simulink model "SF018A_EotProtn"  (R2013b)
settings: Solver=FixedStepDiscrete  SolverMode=SingleTasking  StartTime=0.0  StopTime=0.002  FixedStep=.002  RelTol=1e-3
undefined symbols (not defined in the file): ALLSPDDAMPG_CNT_U08, ALLSPDGAIN_CNT_U08, ARCHGLBPRM_2MILLISEC_SEC_F32, DISTLPFILFRQ_HZ_F32, EOTDAMPGLOLIM_MOTNWTMTR_F32, EOTGAINHILIM_ULS_F32, EotProtnActvRegnBypMaxThd, EotProtnDampgSlew, EotProtnDampgVehSpdTbl, EotProtnDeltaTqThd, EotProtnDftPosn, EotProtnEntrGainVehSpdTbl, EotProtnEntrGainX, EotProtnEntrStLpFilFrq, EotProtnExitDampgY, EotProtnExitStLpFilFrq, EotProtnHwAgGain, EotProtnHwAgMax, EotProtnHwAgMin, EotProtnHwDegDampgX, EotProtnMotSpdIncptSca, EotProtnMotSpdIncptX, EotProtnMotSpdIncptY, EotProtnMotVelGain, EotProtnNormDampgY, EotProtnPosnRampStep, EotProtnRackTrvlLimrAuthyThd, EotProtnRackTrvlLimrAuthyThdLimd, EotProtnRackTrvlLimrEna, EotProtnRackTrvlLimrRng, EotProtnRackTrvlLimrRngLimd, EotProtnRackTrvlLimrVehSpdThd, EotProtnRunEotVelImpctAndSoftEndStop, EotProtnSoftEndStopAuthyThd, EotProtnSoftEndStopEna, EotProtnSoftEndStopVehSpdThd, FIRSTPTDAMPG_CNT_U08, LASTPTGAIN_CNT_U08, SOFTENDSTOPSTDI_CNT_U08, SOFTENDSTOPSTENTR_CNT_U08, SOFTENDSTOPSTEXIT_CNT_U08, SOFTENDSTOPSTNORM_CNT_U08, SYSGLBPRM_MOTTQCMDHILIM_MOTNWTMTR_F32, ZEROMOTTQCMD_MOTNWTMTR_F32
libraries: NxtrAbslt x16, FloatToFixd x14, FixdToFloat x6, Fil x5, NxtrLim x5, simulink x4, NxtrMax x4, LnrIntrpnDyn x3, NxtrSign x2, BilnrIntrpnMplXDyn x2, BilnrIntrpnMplX x1, LnrIntrpn x1
(part 4 of 5)

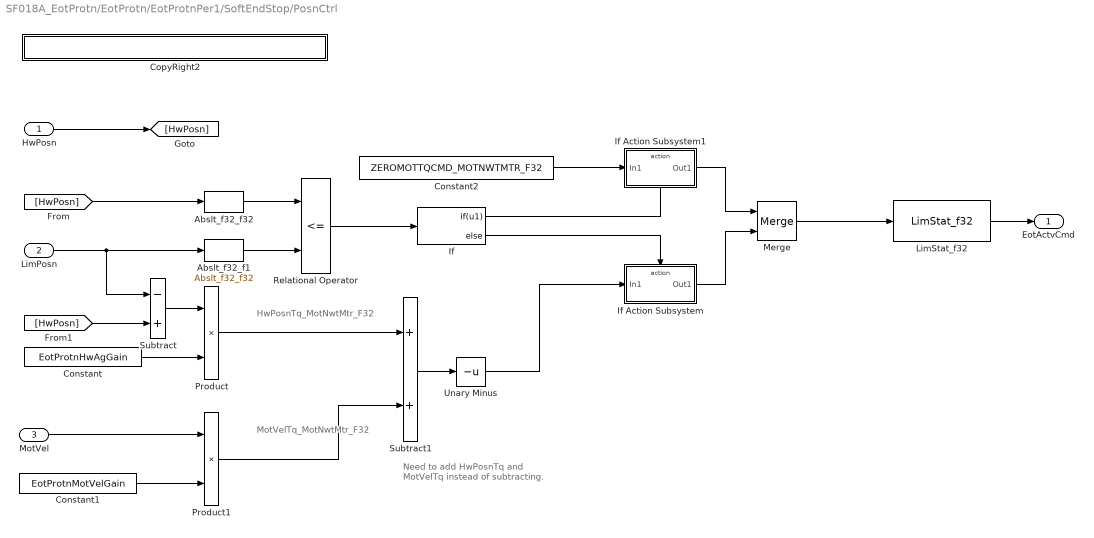
== system SF018A_EotProtn/EotProtn/EotProtnPer1/SoftEndStop/PosnCtrl ==
  note: Need to add HwPosnTq and
      | MotVelTq instead of subtracting.
  note: HwPosnTq_MotNwtMtr_F32
  note: MotVelTq_MotNwtMtr_F32
  HwPosn : Inport
  LimPosn : Inport  Port=2
  MotVel : Inport  Port=3
  Abslt_f32_f1 : NxtrAbslt/Abslt_f32_f32  SFunctionSpec=single y1 = Abslt_f32_f32(single u1)
      settings: AttributesFormatString=%<Name>
  Abslt_f32_f32 : NxtrAbslt/Abslt_f32_f32  SFunctionSpec=single y1 = Abslt_f32_f32(single u1)
      settings: AttributesFormatString=%<Name>
  Constant : Constant  Value=EotProtnHwAgGain
  Constant1 : Constant  Value=EotProtnMotVelGain
  Constant2 : Constant  RequirementInfo={'linktype_rmi_doors' '0000ba56 (/E-STEER Core/SubSystem Specifications/Application Functions/SF018A End-of-Travel Actuator Management- EOT Impact and Soft Stops)' '#SF018A_118' 'true' 'REQ: SF018A_118' '' } %GIDa_3d57071b_fdcd_4c59_a01b_b9a326557455  Value=ZEROMOTTQCMD_MOTNWTMTR_F32
  CopyRight2 : Subsystem  Description=|  mask(Copyright Information){none=on}
      | Copyright info block.                                               
      |                                                                     
      | Place copyright information at the top of every subsystem in design.
      mask prompts: none "No parameters"
      mask help: Place copyright information at the top of every subsystem in design.
      mask Display:
      | NxtrConf = 'Nexteer Confidential';
      | 
      | sys = bdroot; %handle for the current model ("system")
      | first = get_param(sys,'Created');
      | if(isempty(first))
      |     first = datestr(now,'yyyy');
      | else
      |     first = first(end-3:end);  %year is last four digits
      | end
      | 
      | last = get_param(sys,'LastModifiedDate');
      | if isempty(last)
      |     last = datestr(now,'yyyy');
      | else
      |     last = last(end-3:end);
      | end
      | 
      | if strcmp(first,last)
      |     fprintf('%s -- Copyright %s Nexteer',NxtrConf,first)
      | else
      |     fprintf('%s -- %s%s- %s Nexteer',NxtrConf,char(169),first,last)
      | end
  If : If  RequirementInfo={'linktype_rmi_doors' '0000ba56 (/E-STEER Core/SubSystem Specifications/Application Functions/SF018A End-of-Travel Actuator Management- EOT Impact and Soft Stops)' '#SF018A_118' 'true' 'REQ: SF018A_118' '' } %GIDa_eb767372_f633_4e49_a326_b612579dcde1  IfExpression=u1
  If Action Subsystem : Subsystem  RequirementInfo={'linktype_rmi_doors' '0000ba56 (/E-STEER Core/SubSystem Specifications/Application Functions/SF018A End-of-Travel Actuator Management- EOT Impact and Soft Stops)' '#SF018A_118' 'true' 'REQ: SF018A_118' '' } %GIDa_35741698_416e_4048_a750_0a2756a8727b  TreatAsAtomicUnit=on
  If Action Subsystem1 : Subsystem  RequirementInfo={'linktype_rmi_doors' '0000ba56 (/E-STEER Core/SubSystem Specifications/Application Functions/SF018A End-of-Travel Actuator Management- EOT Impact and Soft Stops)' '#SF018A_118' 'true' 'REQ: SF018A_118' '' } %GIDa_3f03eff5_f878_4981_ae49_8a66d8cca778  TreatAsAtomicUnit=on
  LimStat_f32 : NxtrLim/LimStat_f32  RequirementInfo={'linktype_rmi_doors' '0000ba56 (/E-STEER Core/SubSystem Specifications/Application Functions/SF018A End-of-Travel Actuator Management- EOT Impact and Soft Stops)' '#SF018A_115' 'true' 'REQ: SF018A_115' '' } %GIDa_f450d0e0_b743_4f7d_a6bc_c122e939de08  LoLim=SYSGLBPRM_MOTTQCMDLOLIM_MOTNWTMTR_F32  HiLim=SYSGLBPRM_MOTTQCMDHILIM_MOTNWTMTR_F32
      settings: AttributesFormatString=|
      | Low Limit: %<LoLim>
      | High Limit:%<HiLim>
  Merge : Merge  RequirementInfo={'linktype_rmi_doors' '0000ba56 (/E-STEER Core/SubSystem Specifications/Application Functions/SF018A End-of-Travel Actuator Management- EOT Impact and Soft Stops)' '#SF018A_118' 'true' 'REQ: SF018A_118' '' } %GIDa_35b0fcf4_10cf_4d00_afb1_7de2ceba647a
  Product : Product  RequirementInfo={'linktype_rmi_doors' '0000ba56 (/E-STEER Core/SubSystem Specifications/Application Functions/SF018A End-of-Travel Actuator Management- EOT Impact and Soft Stops)' '#SF018A_115' 'true' 'REQ: SF018A_115' '' } %GIDa_75e8deb4_4dc3_4dee_b8fd_971ee3dd6133
  Product1 : Product  RequirementInfo={'linktype_rmi_doors' '0000ba56 (/E-STEER Core/SubSystem Specifications/Application Functions/SF018A End-of-Travel Actuator Management- EOT Impact and Soft Stops)' '#SF018A_115' 'true' 'REQ: SF018A_115' '' } %GIDa_7846ba9c_06f8_474a_b2f4_81c28a29a3d7
  Relational Operator : RelationalOperator  RequirementInfo={'linktype_rmi_doors' '0000ba56 (/E-STEER Core/SubSystem Specifications/Application Functions/SF018A End-of-Travel Actuator Management- EOT Impact and Soft Stops)' '#SF018A_118' 'true' 'REQ: SF018A_118' '' } %GIDa_f3de5d6e_d215_4d21_9e68_558719ac5ade  Operator=<=  OutDataTypeStr=boolean
  Subtract : Sum  RequirementInfo={'linktype_rmi_doors' '0000ba56 (/E-STEER Core/SubSystem Specifications/Application Functions/SF018A End-of-Travel Actuator Management- EOT Impact and Soft Stops)' '#SF018A_115' 'true' 'REQ: SF018A_115' '' } %GIDa_15a4990c_45d6_482c_b0b5_8f5c16105016  Inputs=-+
  Subtract1 : Sum  RequirementInfo={'linktype_rmi_doors' '0000ba56 (/E-STEER Core/SubSystem Specifications/Application Functions/SF018A End-of-Travel Actuator Management- EOT Impact and Soft Stops)' '#SF018A_116' 'true' 'REQ: SF018A_116' '' ; 'linktype_rmi_doors' '0000ba56 (/E-STEER Core/SubSystem Specifications/Application Functions/SF018A End-of-Travel Actuator Management- EOT Impact and Soft Stops)' '#SF018A_117' 'true' 'REQ: SF018A_117' '' } %GIDa_cd110dc1_ef6c_4228_8a84_7b55c0e467bf
  Unary Minus : UnaryMinus
  EotActvCmd : Outport
  wires:
  Unary Minus/1 -> If Action Subsystem/1(In1)
  LimStat_f32/1 -> EotActvCmd/1
  Merge/1 -> LimStat_f32/1
  If Action Subsystem/1(Out1) -> Merge/2
  If Action Subsystem1/1(Out1) -> Merge/1
  Constant2/1 -> If Action Subsystem1/1(In1)
  If/1 -> If Action Subsystem1/Action
  If/2 -> If Action Subsystem/Action
  Subtract1/1 -> Unary Minus/1
  Relational Operator/1 -> If/1
  Abslt_f32_f1/1 -> Relational Operator/2
  Abslt_f32_f32/1 -> Relational Operator/1
  Constant1/1 -> Product1/2
  MotVel/1 -> Product1/1
  Product1/1 -> Subtract1/2
  Constant/1 -> Product/2
  [HwPosn] -> Subtract/2
  LimPosn/1 -> Abslt_f32_f1/1, Subtract/1
  [HwPosn] -> Abslt_f32_f32/1
  HwPosn/1 -> [HwPosn]
  Subtract/1 -> Product/1
  Product/1 -> Subtract1/1

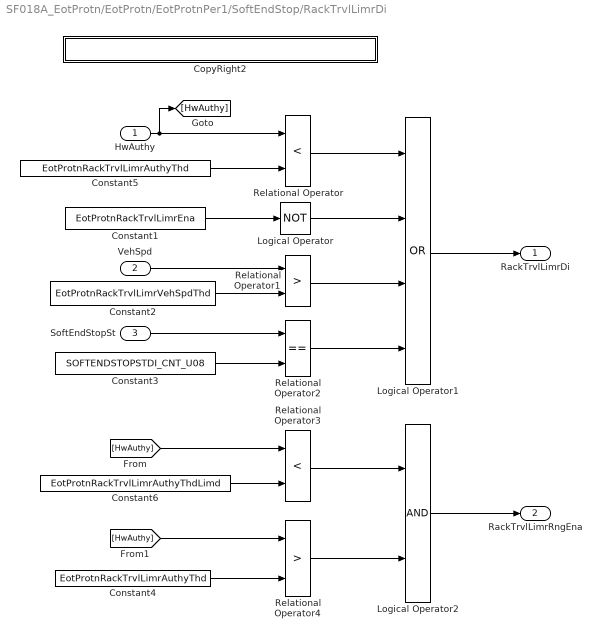
== system SF018A_EotProtn/EotProtn/EotProtnPer1/SoftEndStop/RackTrvlLimrDi ==
  HwAuthy : Inport
  VehSpd : Inport  Port=2
  SoftEndStopSt : Inport  Port=3
  Constant1 : Constant  RequirementInfo={'linktype_rmi_doors' '0000ba56 (/E-STEER Core/SubSystem Specifications/Application Functions/SF018A End-of-Travel Actuator Management- EOT Impact and Soft Stops)' '#SF018A_120' 'true' 'REQ: SF018A_120' '' } %GIDa_59740265_ba46_45fa_b542_907847063bc8  Value=EotProtnRackTrvlLimrEna
  Constant2 : Constant  RequirementInfo={'linktype_rmi_doors' '0000ba56 (/E-STEER Core/SubSystem Specifications/Application Functions/SF018A End-of-Travel Actuator Management- EOT Impact and Soft Stops)' '#SF018A_119' 'true' 'REQ: SF018A_119' '' } %GIDa_beb46b93_86dd_47fa_b05d_730f56507c38  Value=EotProtnRackTrvlLimrVehSpdThd
  Constant3 : Constant  Value=SOFTENDSTOPSTDI_CNT_U08
  Constant4 : Constant  RequirementInfo={'linktype_rmi_doors' '0000ba56 (/E-STEER Core/SubSystem Specifications/Application Functions/SF018A End-of-Travel Actuator Management- EOT Impact and Soft Stops)' '#SF018A_171' 'true' 'REQ: SF018A_171' '' } %GIDa_495d48d6_8769_4499_938f_3fc14f788b0f  Value=EotProtnRackTrvlLimrAuthyThd
  Constant5 : Constant  RequirementInfo={'linktype_rmi_doors' '0000ba56 (/E-STEER Core/SubSystem Specifications/Application Functions/SF018A End-of-Travel Actuator Management- EOT Impact and Soft Stops)' '#SF018A_118' 'true' 'REQ: SF018A_118' '' } %GIDa_b6a052ed_1605_41df_905d_0f8919a88f08  Value=EotProtnRackTrvlLimrAuthyThd
  Constant6 : Constant  RequirementInfo={'linktype_rmi_doors' '0000ba56 (/E-STEER Core/SubSystem Specifications/Application Functions/SF018A End-of-Travel Actuator Management- EOT Impact and Soft Stops)' '#SF018A_171' 'true' 'REQ: SF018A_171' '' } %GIDa_950032d3_08de_4546_a354_35ebe8f18f56  Value=EotProtnRackTrvlLimrAuthyThdLimd
  CopyRight2 : Subsystem  Description=|  mask(Copyright Information){none=on}
      | Copyright info block.                                               
      |                                                                     
      | Place copyright information at the top of every subsystem in design.
      mask prompts: none "No parameters"
      mask help: Place copyright information at the top of every subsystem in design.
      mask Display:
      | NxtrConf = 'Nexteer Confidential';
      | 
      | sys = bdroot; %handle for the current model ("system")
      | first = get_param(sys,'Created');
      | if(isempty(first))
      |     first = datestr(now,'yyyy');
      | else
      |     first = first(end-3:end);  %year is last four digits
      | end
      | 
      | last = get_param(sys,'LastModifiedDate');
      | if isempty(last)
      |     last = datestr(now,'yyyy');
      | else
      |     last = last(end-3:end);
      | end
      | 
      | if strcmp(first,last)
      |     fprintf('%s -- Copyright %s Nexteer',NxtrConf,first)
      | else
      |     fprintf('%s -- %s%s- %s Nexteer',NxtrConf,char(169),first,last)
      | end
  Logical Operator : Logic  RequirementInfo={'linktype_rmi_doors' '0000ba56 (/E-STEER Core/SubSystem Specifications/Application Functions/SF018A End-of-Travel Actuator Management- EOT Impact and Soft Stops)' '#SF018A_120' 'true' 'REQ: SF018A_120' '' } %GIDa_993b19eb_132f_4bd7_8614_13ffb579c74a  Operator=NOT  Inputs=1  AllPortsSameDT=off  OutDataTypeStr=boolean
  Logical Operator1 : Logic  RequirementInfo={'linktype_rmi_doors' '0000ba56 (/E-STEER Core/SubSystem Specifications/Application Functions/SF018A End-of-Travel Actuator Management- EOT Impact and Soft Stops)' '#SF018A_118' 'true' 'REQ: SF018A_118' '' ; 'linktype_rmi_doors' '0000ba56 (/E-STEER Core/SubSystem Specifications/Application Functions/SF018A End-of-Travel Actuator Management- EOT Impact and Soft Stops)' '#SF018A_119' 'true' 'REQ: SF018A_119' '' ; 'linktype_rmi_doors' '0000ba56 (/E-STEER Core/SubSystem Specifications/Application Functions/SF018A End-of-Travel Actuator Management- EOT Impact and Soft Stops)' '#SF018A_120' 'true' 'REQ: SF018A_120' '' } %GIDa_634adabe_71c4_477a_9d97_af2c9c129803  Operator=OR  Inputs=4  AllPortsSameDT=off  OutDataTypeStr=boolean
  Logical Operator2 : Logic  RequirementInfo={'linktype_rmi_doors' '0000ba56 (/E-STEER Core/SubSystem Specifications/Application Functions/SF018A End-of-Travel Actuator Management- EOT Impact and Soft Stops)' '#SF018A_171' 'true' 'REQ: SF018A_171' '' } %GIDa_da8473f5_f718_4aff_af80_eae1cf934d60  AllPortsSameDT=off  OutDataTypeStr=boolean
  Relational Operator : RelationalOperator  RequirementInfo={'linktype_rmi_doors' '0000ba56 (/E-STEER Core/SubSystem Specifications/Application Functions/SF018A End-of-Travel Actuator Management- EOT Impact and Soft Stops)' '#SF018A_118' 'true' 'REQ: SF018A_118' '' } %GIDa_2d353d15_6c28_487c_91b6_406d31ef4a3e  Operator=<  OutDataTypeStr=boolean
  Relational Operator1 : RelationalOperator  RequirementInfo={'linktype_rmi_doors' '0000ba56 (/E-STEER Core/SubSystem Specifications/Application Functions/SF018A End-of-Travel Actuator Management- EOT Impact and Soft Stops)' '#SF018A_119' 'true' 'REQ: SF018A_119' '' } %GIDa_37c960fb_a8f8_4776_adbe_58d92d83a73b  Operator=>  OutDataTypeStr=boolean
  Relational Operator2 : RelationalOperator  Operator===  OutDataTypeStr=boolean
  Relational Operator3 : RelationalOperator  RequirementInfo={'linktype_rmi_doors' '0000ba56 (/E-STEER Core/SubSystem Specifications/Application Functions/SF018A End-of-Travel Actuator Management- EOT Impact and Soft Stops)' '#SF018A_171' 'true' 'REQ: SF018A_171' '' } %GIDa_8979b43c_a751_4f1f_94b9_e7a6732fc66e  Operator=<  OutDataTypeStr=boolean
  Relational Operator4 : RelationalOperator  RequirementInfo={'linktype_rmi_doors' '0000ba56 (/E-STEER Core/SubSystem Specifications/Application Functions/SF018A End-of-Travel Actuator Management- EOT Impact and Soft Stops)' '#SF018A_171' 'true' 'REQ: SF018A_171' '' } %GIDa_92138053_b9f4_4b4b_b437_f353b61a6e67  Operator=>  OutDataTypeStr=boolean
  RackTrvlLimrDi : Outport
  RackTrvlLimrRngEna : Outport  RequirementInfo={'linktype_rmi_doors' '0000ba56 (/E-STEER Core/SubSystem Specifications/Application Functions/SF018A End-of-Travel Actuator Management- EOT Impact and Soft Stops)' '#SF018A_171' 'true' 'REQ: SF018A_171' '' } %GIDa_517743c5_28d1_4dae_83fb_b0af30e05223  Port=2
  wires:
  Logical Operator1/1 -> RackTrvlLimrDi/1
  Relational Operator2/1 -> Logical Operator1/4
  Relational Operator/1 -> Logical Operator1/1
  Logical Operator/1 -> Logical Operator1/2
  Relational Operator1/1 -> Logical Operator1/3
  Constant3/1 -> Relational Operator2/2
  SoftEndStopSt/1 -> Relational Operator2/1
  Constant2/1 -> Relational Operator1/2
  VehSpd/1 -> Relational Operator1/1
  Constant1/1 -> Logical Operator/1
  Constant5/1 -> Relational Operator/2
  HwAuthy/1 -> [HwAuthy], Relational Operator/1
  [HwAuthy] -> Relational Operator3/1
  [HwAuthy] -> Relational Operator4/1
  Relational Operator3/1 -> Logical Operator2/1
  Relational Operator4/1 -> Logical Operator2/2
  Logical Operator2/1 -> RackTrvlLimrRngEna/1
  Constant4/1 -> Relational Operator4/2
  Constant6/1 -> Relational Operator3/2

== system SF018A_EotProtn/EotProtn/EotProtnPer1/SoftEndStop/RackTrvlLimrInin ==
  note: NOT and AND blocks have been removed from here
  note: False
  note: True
  RackTrvlLimrDi : Inport
  HwPosn : Inport  Port=2
  LimPosn : Inport  Port=3
  Abslt_f32_f1 : NxtrAbslt/Abslt_f32_f32  RequirementInfo={'linktype_rmi_doors' '0000ba56 (/E-STEER Core/SubSystem Specifications/Application Functions/SF018A End-of-Travel Actuator Management- EOT Impact and Soft Stops)' '#SF018A_149' 'true' 'REQ: SF018A_149' '' ; 'linktype_rmi_doors' '0000ba56 (/E-STEER Core/SubSystem Specifications/Application Functions/SF018A End-of-Travel Actuator Management- EOT Impact and Soft Stops)' '#SF018A_154' 'true' 'REQ: SF018A_154' '' } %GIDa_9c6107c5_1c8e_4683_9408_653d7285d7d9  SFunctionSpec=single y1 = Abslt_f32_f32(single u1)
      settings: AttributesFormatString=%<Name>
  Abslt_f32_f32 : NxtrAbslt/Abslt_f32_f32  RequirementInfo={'linktype_rmi_doors' '0000ba56 (/E-STEER Core/SubSystem Specifications/Application Functions/SF018A End-of-Travel Actuator Management- EOT Impact and Soft Stops)' '#SF018A_149' 'true' 'REQ: SF018A_149' '' ; 'linktype_rmi_doors' '0000ba56 (/E-STEER Core/SubSystem Specifications/Application Functions/SF018A End-of-Travel Actuator Management- EOT Impact and Soft Stops)' '#SF018A_154' 'true' 'REQ: SF018A_154' '' } %GIDa_808a6b83_c1c0_432d_bdb8_cd3754f3cc18  SFunctionSpec=single y1 = Abslt_f32_f32(single u1)
      settings: AttributesFormatString=%<Name>
  CopyRight2 : Subsystem  Description=|  mask(Copyright Information){none=on}
      | Copyright info block.                                               
      |                                                                     
      | Place copyright information at the top of every subsystem in design.
      mask prompts: none "No parameters"
      mask help: Place copyright information at the top of every subsystem in design.
      mask Display:
      | NxtrConf = 'Nexteer Confidential';
      | 
      | sys = bdroot; %handle for the current model ("system")
      | first = get_param(sys,'Created');
      | if(isempty(first))
      |     first = datestr(now,'yyyy');
      | else
      |     first = first(end-3:end);  %year is last four digits
      | end
      | 
      | last = get_param(sys,'LastModifiedDate');
      | if isempty(last)
      |     last = datestr(now,'yyyy');
      | else
      |     last = last(end-3:end);
      | end
      | 
      | if strcmp(first,last)
      |     fprintf('%s -- Copyright %s Nexteer',NxtrConf,first)
      | else
      |     fprintf('%s -- %s%s- %s Nexteer',NxtrConf,char(169),first,last)
      | end
  Data Store Read : DataStoreRead  RequirementInfo={'linktype_rmi_doors' '0000ba56 (/E-STEER Core/SubSystem Specifications/Application Functions/SF018A End-of-Travel Actuator Management- EOT Impact and Soft Stops)' '#SF018A_152' 'true' 'REQ: SF018A_152' '' } %GIDa_327edd3f_b19e_465c_9235_e27b1a8cba8c  DataStoreName=PrevRackTrvlLimrInin
  If : If  RequirementInfo={'linktype_rmi_doors' '0000ba56 (/E-STEER Core/SubSystem Specifications/Application Functions/SF018A End-of-Travel Actuator Management- EOT Impact and Soft Stops)' '#SF018A_126' 'true' 'REQ: SF018A_126' '' ; 'linktype_rmi_doors' '0000ba56 (/E-STEER Core/SubSystem Specifications/Application Functions/SF018A End-of-Travel Actuator Management- EOT Impact and Soft Stops)' '#SF018A_129' 'true' 'REQ: SF018A_129' '' } %GIDa_41971605_daa9_4a9b_afa4_b65adca64da7  NumInputs=2  IfExpression=u1  ElseIfExpressions=u2
  If Action Subsystem : Subsystem  TreatAsAtomicUnit=on
  If Action Subsystem1 : Subsystem  RequirementInfo={} %GIDa_4c8ec6ee_c625_4bfd_b5dc_d910733b75e9  TreatAsAtomicUnit=on
  If Action Subsystem2 : Subsystem  RequirementInfo={'linktype_rmi_doors' '0000ba56 (/E-STEER Core/SubSystem Specifications/Application Functions/SF018A End-of-Travel Actuator Management- EOT Impact and Soft Stops)' '#SF018A_152' 'true' 'REQ: SF018A_152' '' } %GIDa_b0a0ba46_4120_4f90_926f_e83605afeb20  TreatAsAtomicUnit=on
  Merge2 : Merge  RequirementInfo={'linktype_rmi_doors' '0000ba56 (/E-STEER Core/SubSystem Specifications/Application Functions/SF018A End-of-Travel Actuator Management- EOT Impact and Soft Stops)' '#SF018A_126' 'true' 'REQ: SF018A_126' '' ; 'linktype_rmi_doors' '0000ba56 (/E-STEER Core/SubSystem Specifications/Application Functions/SF018A End-of-Travel Actuator Management- EOT Impact and Soft Stops)' '#SF018A_129' 'true' 'REQ: SF018A_129' '' } %GIDa_56cc687d_545c_452c_a8cf_703dac935b33  Inputs=3
  Relational Operator3 : RelationalOperator  RequirementInfo={'linktype_rmi_doors' '0000ba56 (/E-STEER Core/SubSystem Specifications/Application Functions/SF018A End-of-Travel Actuator Management- EOT Impact and Soft Stops)' '#SF018A_124' 'true' 'REQ: SF018A_124' '' ; 'linktype_rmi_doors' '0000ba56 (/E-STEER Core/SubSystem Specifications/Application Functions/SF018A End-of-Travel Actuator Management- EOT Impact and Soft Stops)' '#SF018A_129' 'true' 'REQ: SF018A_129' '' ; 'linktype_rmi_doors' '0000ba56 (/E-STEER Core/SubSystem Specifications/Application Functions/SF018A End-of-Travel Actuator Management- EOT Impact and Soft Stops)' '#SF018A_130' 'true' 'REQ: SF018A_130' '' ; 'linktype_rmi_doors' '0000ba56 (/E-STEER Core/SubSystem Specifications/Application Functions/SF018A End-of-Travel Actuator Management- EOT Impact and Soft Stops)' '#SF018A_153' 'true' 'REQ: SF018A_153' '' } %GIDa_641eaaa3_1c37_44b9_995f_5dcf0be74e8e  Operator=<=  OutDataTypeStr=boolean
  RackTrvlLimrInin : Outport
  wires:
  Data Store Read/1 -> If Action Subsystem2/1(In1)
  Merge2/1 -> RackTrvlLimrInin/1
  If/3 -> If Action Subsystem2/Action
  If/2 -> If Action Subsystem1/Action
  If/1 -> If Action Subsystem/Action
  If Action Subsystem2/1(Out1) -> Merge2/3
  If Action Subsystem1/1(false) -> Merge2/2
  If Action Subsystem/1(true) -> Merge2/1
  RackTrvlLimrDi/1 -> If/2
  Relational Operator3/1 -> If/1
  Abslt_f32_f32/1 -> Relational Operator3/1
  Abslt_f32_f1/1 -> Relational Operator3/2
  LimPosn/1 -> Abslt_f32_f1/1
  HwPosn/1 -> Abslt_f32_f32/1

== system SF018A_EotProtn/EotProtn/EotProtnPer1/SoftEndStopStCtrl/CopyRight2 ==

== system SF018A_EotProtn/EotProtn/EotProtnPer1/SoftEndStopStCtrl/Keep State ==
  In1 : Inport
  Action Port : ActionPort  ActionType=else
  CopyRight2 : Subsystem  Description=|  mask(Copyright Information){none=on}
      | Copyright info block.                                               
      |                                                                     
      | Place copyright information at the top of every subsystem in design.
      mask prompts: none "No parameters"
      mask help: Place copyright information at the top of every subsystem in design.
      mask Display:
      | NxtrConf = 'Nexteer Confidential';
      | 
      | sys = bdroot; %handle for the current model ("system")
      | first = get_param(sys,'Created');
      | if(isempty(first))
      |     first = datestr(now,'yyyy');
      | else
      |     first = first(end-3:end);  %year is last four digits
      | end
      | 
      | last = get_param(sys,'LastModifiedDate');
      | if isempty(last)
      |     last = datestr(now,'yyyy');
      | else
      |     last = last(end-3:end);
      | end
      | 
      | if strcmp(first,last)
      |     fprintf('%s -- Copyright %s Nexteer',NxtrConf,first)
      | else
      |     fprintf('%s -- %s%s- %s Nexteer',NxtrConf,char(169),first,last)
      | end
  Out1 : Outport
  wires:
  In1/1 -> Out1/1

== system SF018A_EotProtn/EotProtn/EotProtnPer1/SoftEndStopStCtrl/PriorityVec1 ==
  In1 : Inport
  Action Port : ActionPort  ActionType=then
  CopyRight2 : Subsystem  Description=|  mask(Copyright Information){none=on}
      | Copyright info block.                                               
      |                                                                     
      | Place copyright information at the top of every subsystem in design.
      mask prompts: none "No parameters"
      mask help: Place copyright information at the top of every subsystem in design.
      mask Display:
      | NxtrConf = 'Nexteer Confidential';
      | 
      | sys = bdroot; %handle for the current model ("system")
      | first = get_param(sys,'Created');
      | if(isempty(first))
      |     first = datestr(now,'yyyy');
      | else
      |     first = first(end-3:end);  %year is last four digits
      | end
      | 
      | last = get_param(sys,'LastModifiedDate');
      | if isempty(last)
      |     last = datestr(now,'yyyy');
      | else
      |     last = last(end-3:end);
      | end
      | 
      | if strcmp(first,last)
      |     fprintf('%s -- Copyright %s Nexteer',NxtrConf,first)
      | else
      |     fprintf('%s -- %s%s- %s Nexteer',NxtrConf,char(169),first,last)
      | end
  Out1 : Outport
  wires:
  In1/1 -> Out1/1

== system SF018A_EotProtn/EotProtn/EotProtnPer1/SoftEndStopStCtrl/PriorityVec2 ==
  In1 : Inport
  Action Port : ActionPort  ActionType=elseif
  CopyRight2 : Subsystem  Description=|  mask(Copyright Information){none=on}
      | Copyright info block.                                               
      |                                                                     
      | Place copyright information at the top of every subsystem in design.
      mask prompts: none "No parameters"
      mask help: Place copyright information at the top of every subsystem in design.
      mask Display:
      | NxtrConf = 'Nexteer Confidential';
      | 
      | sys = bdroot; %handle for the current model ("system")
      | first = get_param(sys,'Created');
      | if(isempty(first))
      |     first = datestr(now,'yyyy');
      | else
      |     first = first(end-3:end);  %year is last four digits
      | end
      | 
      | last = get_param(sys,'LastModifiedDate');
      | if isempty(last)
      |     last = datestr(now,'yyyy');
      | else
      |     last = last(end-3:end);
      | end
      | 
      | if strcmp(first,last)
      |     fprintf('%s -- Copyright %s Nexteer',NxtrConf,first)
      | else
      |     fprintf('%s -- %s%s- %s Nexteer',NxtrConf,char(169),first,last)
      | end
  Out1 : Outport
  wires:
  In1/1 -> Out1/1

== system SF018A_EotProtn/EotProtn/EotProtnPer1/SoftEndStopStCtrl/PriorityVec3 ==
  In1 : Inport
  Action Port : ActionPort  ActionType=elseif
  CopyRight2 : Subsystem  Description=|  mask(Copyright Information){none=on}
      | Copyright info block.                                               
      |                                                                     
      | Place copyright information at the top of every subsystem in design.
      mask prompts: none "No parameters"
      mask help: Place copyright information at the top of every subsystem in design.
      mask Display:
      | NxtrConf = 'Nexteer Confidential';
      | 
      | sys = bdroot; %handle for the current model ("system")
      | first = get_param(sys,'Created');
      | if(isempty(first))
      |     first = datestr(now,'yyyy');
      | else
      |     first = first(end-3:end);  %year is last four digits
      | end
      | 
      | last = get_param(sys,'LastModifiedDate');
      | if isempty(last)
      |     last = datestr(now,'yyyy');
      | else
      |     last = last(end-3:end);
      | end
      | 
      | if strcmp(first,last)
      |     fprintf('%s -- Copyright %s Nexteer',NxtrConf,first)
      | else
      |     fprintf('%s -- %s%s- %s Nexteer',NxtrConf,char(169),first,last)
      | end
  Out1 : Outport
  wires:
  In1/1 -> Out1/1

== system SF018A_EotProtn/EotProtn/EotProtnPer1/SoftEndStopStCtrl/PriorityVec4 ==
  In1 : Inport
  Action Port : ActionPort  ActionType=elseif
  CopyRight2 : Subsystem  Description=|  mask(Copyright Information){none=on}
      | Copyright info block.                                               
      |                                                                     
      | Place copyright information at the top of every subsystem in design.
      mask prompts: none "No parameters"
      mask help: Place copyright information at the top of every subsystem in design.
      mask Display:
      | NxtrConf = 'Nexteer Confidential';
      | 
      | sys = bdroot; %handle for the current model ("system")
      | first = get_param(sys,'Created');
      | if(isempty(first))
      |     first = datestr(now,'yyyy');
      | else
      |     first = first(end-3:end);  %year is last four digits
      | end
      | 
      | last = get_param(sys,'LastModifiedDate');
      | if isempty(last)
      |     last = datestr(now,'yyyy');
      | else
      |     last = last(end-3:end);
      | end
      | 
      | if strcmp(first,last)
      |     fprintf('%s -- Copyright %s Nexteer',NxtrConf,first)
      | else
      |     fprintf('%s -- %s%s- %s Nexteer',NxtrConf,char(169),first,last)
      | end
  Out1 : Outport
  wires:
  In1/1 -> Out1/1

== system SF018A_EotProtn/EotProtn/EotProtnPer1/EotVelImpct/If Action Subsystem/CopyRight2 ==

== system SF018A_EotProtn/EotProtn/EotProtnPer1/EotVelImpct/If Action Subsystem1/CopyRight2 ==

== system SF018A_EotProtn/EotProtn/EotProtnPer1/EotVelImpct/If Action Subsystem2/CopyRight2 ==

== system SF018A_EotProtn/EotProtn/EotProtnPer1/EotVelImpct/If Action Subsystem3/CopyRight2 ==

== system SF018A_EotProtn/EotProtn/EotProtnPer1/EotVelImpct/If Action Subsystem4/CopyRight2 ==

== system SF018A_EotProtn/EotProtn/EotProtnPer1/EotVelImpct/If Action Subsystem5/CopyRight2 ==

== system SF018A_EotProtn/EotProtn/EotProtnPer1/EotVelImpct/Ramp/CopyRight2 ==

== system SF018A_EotProtn/EotProtn/EotProtnPer1/EotVelImpct/Ramp/If Action Subsystem ==
  In1 : Inport
  Action Port : ActionPort  ActionType=else
  CopyRight2 : Subsystem  Description=|  mask(Copyright Information){none=on}
      | Copyright info block.                                               
      |                                                                     
      | Place copyright information at the top of every subsystem in design.
      mask prompts: none "No parameters"
      mask help: Place copyright information at the top of every subsystem in design.
      mask Display:
      | NxtrConf = 'Nexteer Confidential';
      | 
      | sys = bdroot; %handle for the current model ("system")
      | first = get_param(sys,'Created');
      | if(isempty(first))
      |     first = datestr(now,'yyyy');
      | else
      |     first = first(end-3:end);  %year is last four digits
      | end
      | 
      | last = get_param(sys,'LastModifiedDate');
      | if isempty(last)
      |     last = datestr(now,'yyyy');
      | else
      |     last = last(end-3:end);
      | end
      | 
      | if strcmp(first,last)
      |     fprintf('%s -- Copyright %s Nexteer',NxtrConf,first)
      | else
      |     fprintf('%s -- %s%s- %s Nexteer',NxtrConf,char(169),first,last)
      | end
  Out1 : Outport
  wires:
  In1/1 -> Out1/1

== system SF018A_EotProtn/EotProtn/EotProtnPer1/EotVelImpct/Ramp/If Action Subsystem1 ==
  In1 : Inport
  Action Port : ActionPort  ActionType=then
  CopyRight2 : Subsystem  Description=|  mask(Copyright Information){none=on}
      | Copyright info block.                                               
      |                                                                     
      | Place copyright information at the top of every subsystem in design.
      mask prompts: none "No parameters"
      mask help: Place copyright information at the top of every subsystem in design.
      mask Display:
      | NxtrConf = 'Nexteer Confidential';
      | 
      | sys = bdroot; %handle for the current model ("system")
      | first = get_param(sys,'Created');
      | if(isempty(first))
      |     first = datestr(now,'yyyy');
      | else
      |     first = first(end-3:end);  %year is last four digits
      | end
      | 
      | last = get_param(sys,'LastModifiedDate');
      | if isempty(last)
      |     last = datestr(now,'yyyy');
      | else
      |     last = last(end-3:end);
      | end
      | 
      | if strcmp(first,last)
      |     fprintf('%s -- Copyright %s Nexteer',NxtrConf,first)
      | else
      |     fprintf('%s -- %s%s- %s Nexteer',NxtrConf,char(169),first,last)
      | end
  Out1 : Outport
  wires:
  In1/1 -> Out1/1

== system SF018A_EotProtn/EotProtn/EotProtnPer1/SoftEndStop/CalcEntrGain/CopyRight2 ==

== system SF018A_EotProtn/EotProtn/EotProtnPer1/SoftEndStop/CalcEntrGain/If Action Subsystem ==
  In1 : Inport
  Action Port : ActionPort  ActionType=else
  CopyRight2 : Subsystem  Description=|  mask(Copyright Information){none=on}
      | Copyright info block.                                               
      |                                                                     
      | Place copyright information at the top of every subsystem in design.
      mask prompts: none "No parameters"
      mask help: Place copyright information at the top of every subsystem in design.
      mask Display:
      | NxtrConf = 'Nexteer Confidential';
      | 
      | sys = bdroot; %handle for the current model ("system")
      | first = get_param(sys,'Created');
      | if(isempty(first))
      |     first = datestr(now,'yyyy');
      | else
      |     first = first(end-3:end);  %year is last four digits
      | end
      | 
      | last = get_param(sys,'LastModifiedDate');
      | if isempty(last)
      |     last = datestr(now,'yyyy');
      | else
      |     last = last(end-3:end);
      | end
      | 
      | if strcmp(first,last)
      |     fprintf('%s -- Copyright %s Nexteer',NxtrConf,first)
      | else
      |     fprintf('%s -- %s%s- %s Nexteer',NxtrConf,char(169),first,last)
      | end
  Out1 : Outport
  wires:
  In1/1 -> Out1/1

== system SF018A_EotProtn/EotProtn/EotProtnPer1/SoftEndStop/CalcEntrGain/If Action Subsystem1 ==
  In1 : Inport
  Action Port : ActionPort  ActionType=then
  CopyRight2 : Subsystem  Description=|  mask(Copyright Information){none=on}
      | Copyright info block.                                               
      |                                                                     
      | Place copyright information at the top of every subsystem in design.
      mask prompts: none "No parameters"
      mask help: Place copyright information at the top of every subsystem in design.
      mask Display:
      | NxtrConf = 'Nexteer Confidential';
      | 
      | sys = bdroot; %handle for the current model ("system")
      | first = get_param(sys,'Created');
      | if(isempty(first))
      |     first = datestr(now,'yyyy');
      | else
      |     first = first(end-3:end);  %year is last four digits
      | end
      | 
      | last = get_param(sys,'LastModifiedDate');
      | if isempty(last)
      |     last = datestr(now,'yyyy');
      | else
      |     last = last(end-3:end);
      | end
      | 
      | if strcmp(first,last)
      |     fprintf('%s -- Copyright %s Nexteer',NxtrConf,first)
      | else
      |     fprintf('%s -- %s%s- %s Nexteer',NxtrConf,char(169),first,last)
      | end
  Out1 : Outport
  wires:
  In1/1 -> Out1/1

== system SF018A_EotProtn/EotProtn/EotProtnPer1/SoftEndStop/CalcEotDampg/ Disabled ==
  Action Port : ActionPort  ActionType=case
  Constant2 : Constant  Value=EOTDAMPGLOLIM_MOTNWTMTR_F32
  CopyRight2 : Subsystem  Description=|  mask(Copyright Information){none=on}
      | Copyright info block.                                               
      |                                                                     
      | Place copyright information at the top of every subsystem in design.
      mask prompts: none "No parameters"
      mask help: Place copyright information at the top of every subsystem in design.
      mask Display:
      | NxtrConf = 'Nexteer Confidential';
      | 
      | sys = bdroot; %handle for the current model ("system")
      | first = get_param(sys,'Created');
      | if(isempty(first))
      |     first = datestr(now,'yyyy');
      | else
      |     first = first(end-3:end);  %year is last four digits
      | end
      | 
      | last = get_param(sys,'LastModifiedDate');
      | if isempty(last)
      |     last = datestr(now,'yyyy');
      | else
      |     last = last(end-3:end);
      | end
      | 
      | if strcmp(first,last)
      |     fprintf('%s -- Copyright %s Nexteer',NxtrConf,first)
      | else
      |     fprintf('%s -- %s%s- %s Nexteer',NxtrConf,char(169),first,last)
      | end
  DampgLoLim : Outport
  wires:
  Constant2/1 -> DampgLoLim/1

== system SF018A_EotProtn/EotProtn/EotProtnPer1/SoftEndStop/CalcEotDampg/ Exiting ==
  note: Wait for Price Tools
  HwPosn : Inport
  VehSpd : Inport  Port=2
  NewHwDegDampgX : Inport  Port=3
  Action Port : ActionPort  ActionType=case
  Abslt_f32_f32 : NxtrAbslt/Abslt_f32_f32  SFunctionSpec=single y1 = Abslt_f32_f32(single u1)
      settings: AttributesFormatString=%<Name>
  Constant3 : Constant  Value=EotProtnDampgVehSpdTbl
  Constant6 : Constant  Value=EotProtnExitDampgY
  CopyRight2 : Subsystem  Description=|  mask(Copyright Information){none=on}
      | Copyright info block.                                               
      |                                                                     
      | Place copyright information at the top of every subsystem in design.
      mask prompts: none "No parameters"
      mask help: Place copyright information at the top of every subsystem in design.
      mask Display:
      | NxtrConf = 'Nexteer Confidential';
      | 
      | sys = bdroot; %handle for the current model ("system")
      | first = get_param(sys,'Created');
      | if(isempty(first))
      |     first = datestr(now,'yyyy');
      | else
      |     first = first(end-3:end);  %year is last four digits
      | end
      | 
      | last = get_param(sys,'LastModifiedDate');
      | if isempty(last)
      |     last = datestr(now,'yyyy');
      | else
      |     last = last(end-3:end);
      | end
      | 
      | if strcmp(first,last)
      |     fprintf('%s -- Copyright %s Nexteer',NxtrConf,first)
      | else
      |     fprintf('%s -- %s%s- %s Nexteer',NxtrConf,char(169),first,last)
      | end
  ExitEotDampgIncpt : BilnrIntrpnMplXDyn/BilnrIntrpnWithRound_u16_u16MplXu16MplY  RequirementInfo={'linktype_rmi_doors' '0000ba56 (/E-STEER Core/SubSystem Specifications/Application Functions/SF018A End-of-Travel Actuator Management- EOT Impact and Soft Stops)' '#SF018A_112' 'true' 'REQ: SF018A_112' '' } %GIDa_8d0167e4_ccd0_421c_91ec_2c14160d88d0
      settings: AttributesFormatString=Bilnr ( u16MplX , u16MplY )
  FixdToFloat_f32_u16 : FixdToFloat/FixdToFloat_f32_u16  Param1=16
  FloatToFixd_u16_f1 : FloatToFixd/FloatToFixd_u16_f32  Param1=7
  FloatToFixd_u16_f32 : FloatToFixd/FloatToFixd_u16_f32  Param1=4
  EotDampg : Outport
  wires:
  Constant6/1 -> ExitEotDampgIncpt/5
  Constant3/1 -> ExitEotDampgIncpt/3
  NewHwDegDampgX/1 -> ExitEotDampgIncpt/4
  FixdToFloat_f32_u16/1 -> EotDampg/1
  ExitEotDampgIncpt/1 -> FixdToFloat_f32_u16/1
  VehSpd/1 -> FloatToFixd_u16_f1/1
  FloatToFixd_u16_f32/1 -> ExitEotDampgIncpt/1
  FloatToFixd_u16_f1/1 -> ExitEotDampgIncpt/2
  Abslt_f32_f32/1 -> FloatToFixd_u16_f32/1
  HwPosn/1 -> Abslt_f32_f32/1

== system SF018A_EotProtn/EotProtn/EotProtnPer1/SoftEndStop/CalcEotDampg/ Normal OR Entering ==
  HwPosn : Inport
  VehSpd : Inport  Port=2
  NewHwDegDampgX : Inport  Port=3
  Action Port : ActionPort  ActionType=case
  Abslt_f32_f1 : NxtrAbslt/Abslt_f32_f32  SFunctionSpec=single y1 = Abslt_f32_f32(single u1)
      settings: AttributesFormatString=%<Name>
  Constant2 : Constant  Value=EotProtnDampgVehSpdTbl
  Constant4 : Constant  Value=EotProtnNormDampgY
  CopyRight2 : Subsystem  Description=|  mask(Copyright Information){none=on}
      | Copyright info block.                                               
      |                                                                     
      | Place copyright information at the top of every subsystem in design.
      mask prompts: none "No parameters"
      mask help: Place copyright information at the top of every subsystem in design.
      mask Display:
      | NxtrConf = 'Nexteer Confidential';
      | 
      | sys = bdroot; %handle for the current model ("system")
      | first = get_param(sys,'Created');
      | if(isempty(first))
      |     first = datestr(now,'yyyy');
      | else
      |     first = first(end-3:end);  %year is last four digits
      | end
      | 
      | last = get_param(sys,'LastModifiedDate');
      | if isempty(last)
      |     last = datestr(now,'yyyy');
      | else
      |     last = last(end-3:end);
      | end
      | 
      | if strcmp(first,last)
      |     fprintf('%s -- Copyright %s Nexteer',NxtrConf,first)
      | else
      |     fprintf('%s -- %s%s- %s Nexteer',NxtrConf,char(169),first,last)
      | end
  EntrEotDampgIncpt : BilnrIntrpnMplXDyn/BilnrIntrpnWithRound_u16_u16MplXu16MplY  RequirementInfo={'linktype_rmi_doors' '0000ba56 (/E-STEER Core/SubSystem Specifications/Application Functions/SF018A End-of-Travel Actuator Management- EOT Impact and Soft Stops)' '#SF018A_112' 'true' 'REQ: SF018A_112' '' } %GIDa_01ef975f_d3da_440f_8808_af39eb7257d0
      settings: AttributesFormatString=Bilnr ( u16MplX , u16MplY )
  FixdToFloat_f32_u16 : FixdToFloat/FixdToFloat_f32_u16  Param1=16
  FloatToFixd_u16_f1 : FloatToFixd/FloatToFixd_u16_f32  Param1=7
  FloatToFixd_u16_f32 : FloatToFixd/FloatToFixd_u16_f32  Param1=4
  EotDampg : Outport
  wires:
  NewHwDegDampgX/1 -> EntrEotDampgIncpt/4
  HwPosn/1 -> Abslt_f32_f1/1
  FixdToFloat_f32_u16/1 -> EotDampg/1
  EntrEotDampgIncpt/1 -> FixdToFloat_f32_u16/1
  Constant4/1 -> EntrEotDampgIncpt/5
  Constant2/1 -> EntrEotDampgIncpt/3
  FloatToFixd_u16_f1/1 -> EntrEotDampgIncpt/2
  FloatToFixd_u16_f32/1 -> EntrEotDampgIncpt/1
  VehSpd/1 -> FloatToFixd_u16_f1/1
  Abslt_f32_f1/1 -> FloatToFixd_u16_f32/1

== system SF018A_EotProtn/EotProtn/EotProtnPer1/SoftEndStop/CalcEotDampg/CopyRight2 ==

== system SF018A_EotProtn/EotProtn/EotProtnPer1/SoftEndStop/CalcEotDampg/If Action Subsystem ==
  In1 : Inport
  Action Port : ActionPort  ActionType=else
  CopyRight2 : Subsystem  Description=|  mask(Copyright Information){none=on}
      | Copyright info block.                                               
      |                                                                     
      | Place copyright information at the top of every subsystem in design.
      mask prompts: none "No parameters"
      mask help: Place copyright information at the top of every subsystem in design.
      mask Display:
      | NxtrConf = 'Nexteer Confidential';
      | 
      | sys = bdroot; %handle for the current model ("system")
      | first = get_param(sys,'Created');
      | if(isempty(first))
      |     first = datestr(now,'yyyy');
      | else
      |     first = first(end-3:end);  %year is last four digits
      | end
      | 
      | last = get_param(sys,'LastModifiedDate');
      | if isempty(last)
      |     last = datestr(now,'yyyy');
      | else
      |     last = last(end-3:end);
      | end
      | 
      | if strcmp(first,last)
      |     fprintf('%s -- Copyright %s Nexteer',NxtrConf,first)
      | else
      |     fprintf('%s -- %s%s- %s Nexteer',NxtrConf,char(169),first,last)
      | end
  Out1 : Outport
  wires:
  In1/1 -> Out1/1

== system SF018A_EotProtn/EotProtn/EotProtnPer1/SoftEndStop/CalcEotDampg/If Action Subsystem1 ==
  In1 : Inport
  Action Port : ActionPort  ActionType=then
  CopyRight2 : Subsystem  Description=|  mask(Copyright Information){none=on}
      | Copyright info block.                                               
      |                                                                     
      | Place copyright information at the top of every subsystem in design.
      mask prompts: none "No parameters"
      mask help: Place copyright information at the top of every subsystem in design.
      mask Display:
      | NxtrConf = 'Nexteer Confidential';
      | 
      | sys = bdroot; %handle for the current model ("system")
      | first = get_param(sys,'Created');
      | if(isempty(first))
      |     first = datestr(now,'yyyy');
      | else
      |     first = first(end-3:end);  %year is last four digits
      | end
      | 
      | last = get_param(sys,'LastModifiedDate');
      | if isempty(last)
      |     last = datestr(now,'yyyy');
      | else
      |     last = last(end-3:end);
      | end
      | 
      | if strcmp(first,last)
      |     fprintf('%s -- Copyright %s Nexteer',NxtrConf,first)
      | else
      |     fprintf('%s -- %s%s- %s Nexteer',NxtrConf,char(169),first,last)
      | end
  Out1 : Outport
  wires:
  In1/1 -> Out1/1

== system SF018A_EotProtn/EotProtn/EotProtnPer1/SoftEndStop/CalcEotGain/ Disabled ==
  In1 : Inport
  Action Port : ActionPort  ActionType=case
  CopyRight2 : Subsystem  Description=|  mask(Copyright Information){none=on}
      | Copyright info block.                                               
      |                                                                     
      | Place copyright information at the top of every subsystem in design.
      mask prompts: none "No parameters"
      mask help: Place copyright information at the top of every subsystem in design.
      mask Display:
      | NxtrConf = 'Nexteer Confidential';
      | 
      | sys = bdroot; %handle for the current model ("system")
      | first = get_param(sys,'Created');
      | if(isempty(first))
      |     first = datestr(now,'yyyy');
      | else
      |     first = first(end-3:end);  %year is last four digits
      | end
      | 
      | last = get_param(sys,'LastModifiedDate');
      | if isempty(last)
      |     last = datestr(now,'yyyy');
      | else
      |     last = last(end-3:end);
      | end
      | 
      | if strcmp(first,last)
      |     fprintf('%s -- Copyright %s Nexteer',NxtrConf,first)
      | else
      |     fprintf('%s -- %s%s- %s Nexteer',NxtrConf,char(169),first,last)
      | end
  Out1 : Outport
  wires:
  In1/1 -> Out1/1

== system SF018A_EotProtn/EotProtn/EotProtnPer1/SoftEndStop/CalcEotGain/ Exiting ==
  In1 : Inport
  Action Port : ActionPort  ActionType=case
  CopyRight2 : Subsystem  Description=|  mask(Copyright Information){none=on}
      | Copyright info block.                                               
      |                                                                     
      | Place copyright information at the top of every subsystem in design.
      mask prompts: none "No parameters"
      mask help: Place copyright information at the top of every subsystem in design.
      mask Display:
      | NxtrConf = 'Nexteer Confidential';
      | 
      | sys = bdroot; %handle for the current model ("system")
      | first = get_param(sys,'Created');
      | if(isempty(first))
      |     first = datestr(now,'yyyy');
      | else
      |     first = first(end-3:end);  %year is last four digits
      | end
      | 
      | last = get_param(sys,'LastModifiedDate');
      | if isempty(last)
      |     last = datestr(now,'yyyy');
      | else
      |     last = last(end-3:end);
      | end
      | 
      | if strcmp(first,last)
      |     fprintf('%s -- Copyright %s Nexteer',NxtrConf,first)
      | else
      |     fprintf('%s -- %s%s- %s Nexteer',NxtrConf,char(169),first,last)
      | end
  Out1 : Outport
  wires:
  In1/1 -> Out1/1

== system SF018A_EotProtn/EotProtn/EotProtnPer1/SoftEndStop/CalcEotGain/CopyRight2 ==

== system SF018A_EotProtn/EotProtn/EotProtnPer1/SoftEndStop/CalcEotGain/Entering or Normal ==
  In1 : Inport
  Action Port : ActionPort  ActionType=default
  CopyRight2 : Subsystem  Description=|  mask(Copyright Information){none=on}
      | Copyright info block.                                               
      |                                                                     
      | Place copyright information at the top of every subsystem in design.
      mask prompts: none "No parameters"
      mask help: Place copyright information at the top of every subsystem in design.
      mask Display:
      | NxtrConf = 'Nexteer Confidential';
      | 
      | sys = bdroot; %handle for the current model ("system")
      | first = get_param(sys,'Created');
      | if(isempty(first))
      |     first = datestr(now,'yyyy');
      | else
      |     first = first(end-3:end);  %year is last four digits
      | end
      | 
      | last = get_param(sys,'LastModifiedDate');
      | if isempty(last)
      |     last = datestr(now,'yyyy');
      | else
      |     last = last(end-3:end);
      | end
      | 
      | if strcmp(first,last)
      |     fprintf('%s -- Copyright %s Nexteer',NxtrConf,first)
      | else
      |     fprintf('%s -- %s%s- %s Nexteer',NxtrConf,char(169),first,last)
      | end
  Out1 : Outport
  wires:
  In1/1 -> Out1/1

== system SF018A_EotProtn/EotProtn/EotProtnPer1/SoftEndStop/CalcExitGain/CopyRight2 ==

== system SF018A_EotProtn/EotProtn/EotProtnPer1/SoftEndStop/FildEotGain/CopyRight2 ==

== system SF018A_EotProtn/EotProtn/EotProtnPer1/SoftEndStop/FildEotGain/If Action Subsystem3 ==
  In1 : Inport
  Action Port : ActionPort  ActionType=case
  CopyRight2 : Subsystem  Description=|  mask(Copyright Information){none=on}
      | Copyright info block.                                               
      |                                                                     
      | Place copyright information at the top of every subsystem in design.
      mask prompts: none "No parameters"
      mask help: Place copyright information at the top of every subsystem in design.
      mask Display:
      | NxtrConf = 'Nexteer Confidential';
      | 
      | sys = bdroot; %handle for the current model ("system")
      | first = get_param(sys,'Created');
      | if(isempty(first))
      |     first = datestr(now,'yyyy');
      | else
      |     first = first(end-3:end);  %year is last four digits
      | end
      | 
      | last = get_param(sys,'LastModifiedDate');
      | if isempty(last)
      |     last = datestr(now,'yyyy');
      | else
      |     last = last(end-3:end);
      | end
      | 
      | if strcmp(first,last)
      |     fprintf('%s -- Copyright %s Nexteer',NxtrConf,first)
      | else
      |     fprintf('%s -- %s%s- %s Nexteer',NxtrConf,char(169),first,last)
      | end
  Out1 : Outport
  wires:
  In1/1 -> Out1/1
